simulink model "w1p7"  (R2020b)
settings: Solver=VariableStepAuto  StartTime=0.0  StopTime=10.0  RelTol=1e-3
libraries: dspsrcs4 x1
settings Model: Creator=family  LastModifiedBy=family

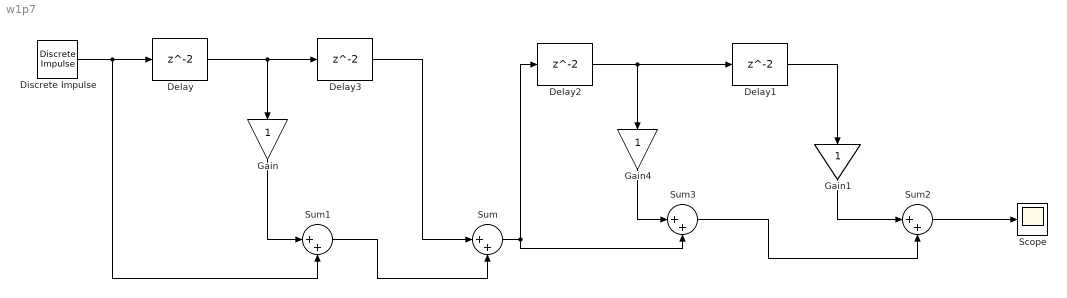
== system w1p7 ==
  Delay{,1..3} (4 alike) : Delay
  Discrete Impulse : dspsrcs4/Discrete  Impulse  Delay=0  SampleTime=1  FrameSample=1  OutputFrames=off  dataType=double  isSigned=on  wordLen=16  udDataType=sfix(16)  fracBitsMode=Best precision  numFracBits=15  OutDataTypeStr=double  LastOutDataTypeStr=double
  Gain : Gain
  Gain1 : Gain
  Gain4 : Gain
  Scope : Scope
  Sum{,1..3} (4 alike) : Sum  Inputs=|++
  wires:
  Delay/1 -> Gain/1, Delay3/1
  Gain/1 -> Sum1/1
  Discrete Impulse/1 -> Sum1/2, Delay/1
  Delay3/1 -> Sum/1
  Sum1/1 -> Sum/2
  Sum/1 -> Delay2/1, Sum3/2
  Delay2/1 -> Delay1/1, Gain4/1
  Gain4/1 -> Sum3/1
  Delay1/1 -> Gain1/1
  Gain1/1 -> Sum2/1
  Sum3/1 -> Sum2/2
  Sum2/1 -> Scope/1
